simulink model "NarmaMotorNoDisrtub"  (R2019b)
settings: Solver=FixedStepAuto  StartTime=0.0  StopTime=30  FixedStep=0.001  RelTol=1e-3
libraries: neural x1, simulink x1
settings Model: Creator=Emanuel  LastModifiedBy=Emanuel

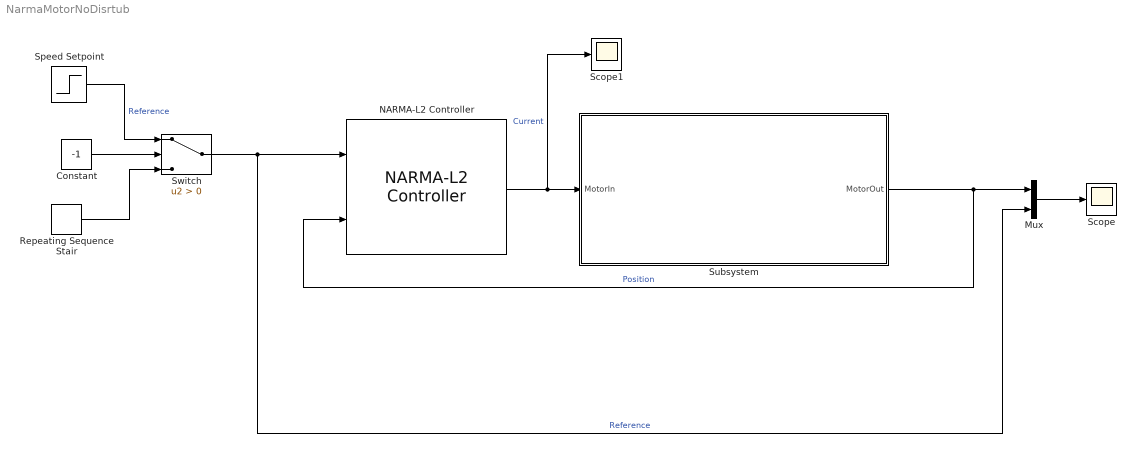
== system NarmaMotorNoDisrtub ==
  Constant : Constant  Value=-1
  Mux : Mux  Inputs=2
  NARMA-L2 Controller : neural/Control Systems/NARMA-L2 Controller  Normalize=0  IW1_1=[0.54422453296791495347 -8.2210065618848435776 -3.7830333244861606978 11.387541350251288108 3.5099764902727077498 -6.615636378792588701 10.270646774195714812 5.4834128974806324308 1.5686929425342031053 1.9741305625561031967 25.064932481428758848;10.05503986873957345 19.028606883106693459 11.182343981242496511 -2.8405339741589590297 -10.464572477682430929 -12.058389281694809725 -2.7714826032906860753 3.7461611803089196471 1.6204644865874766602 0.42415313297564860573 6.4827964395313486534;-335.44078668579430769 286.573015971562711 -187.68734927917793698 319.26608410688868389 221.01642027287860515 -305.40111344708714114 14.276828358611235004 9.9727003878624458366 6.7628793436236751546 9.1349517204525394476 14.179101495100859154;-1.7066174237370790312 -2.2638558722067476658 -2.7406505835762486889 -3.5321189662734870929 -6.5949213353093112389 -14.197286237901327155 2.2799959818071116047 4.0911747950291443843 2.9687832632498922791 3.416878733775998267 5.154880925569540473;-1.6730363884494878768 -5.4151164756102057041 -4.3929057393414607802 -8.1743670020292746869 2.9188688371473987537 18.969447318711061712 -8.529293132078448636 -14.164467720173188781 -10.587852748498855604 -13.551691179760860351 -17.974918470746633403;-3.2591311314982274183 12.337883279114715052 3.2937395594010450139 -30.11284141382879298 32.397534092837638298 -14.32400266854321913 -130.88652771808443731 140.69912550368584903 374.98954455414616405 -459.99858877533671375 -38.476614441129676436]  IW3_2=[-2.7577965784019937701 1.2752231451468867274 1.3996074068349657615 1.2105704890023423204 0.45470321325507695454 -1.2832715227445807837 -0.56158279430395419141 0.37486869307057324452 0.21875572119050948339 0.26450832397968576659 0.77097807764282566545;48.743457576208506055 -5.1531631914190034749 87.065999962059905215 -130.80082279171415394 -103.01087375687944814 97.749403698778010607 71.782150931217856282 55.062621026612909247 42.342961685691626883 43.689160160536054889 47.863257581946839991;5.4573369611260131862 0.22021020308996286374 -24.481423723828033445 -19.157095519588718702 14.135516604963051179 22.874994686256922449 -12.957341738873221715 -3.2165777199510738882 -4.3445828325806790104 -4.4947755060824272633 -3.6135327556077121436;488.07923945828918022 39.889515032705716635 -417.61236881668963861 -624.00642188413860367 371.51404644190978388 122.86999927681219447 -172.9512281008499599 322.0262465292354932 -249.15696488802083763 -274.34942750037879478 -268.53930455658172605;10.614257373293852993 -12.928226038048435953 1.8007341854585847685 0.47590664481989075618 1.3382033156911337102 11.791127023375008065 -1.4570318424168127169 6.6858980619533374679 0.99572516274640121559 3.596724941205785786 5.2562534427693412553;39.573323685332226773 -89.563598565790471184 68.345044595284250022 29.624767071379650929 -64.693171197386988069 16.751714047732363611 9.8626289348993783079 17.769837346136569067 -36.363423331338900368 -48.550247810202122878 -46.730060307809090148]  IW5_3=2.3941954495172454997  LW2_1=[-23.095405534712167395 -2.6857105544596406865 -21.818814964827854652 59.319651534505496215 -14.990739595435632836 11.470481340866285791]  LW4_3=[16.985094766801438482 -4.5039267178616082532 11.682340792277063457 -12.70858501600824475 29.633912642875980481 -6.7500019987399628718]  LW5_4=24.134279084852479969  LW6_5=0.037657415187600851159  LW6_2=-24.147602895572209292  B1=[-4.713627645162457469;-3.0956134780243815818;-958.89880089222197057;0.66118087049018392509;2.3947070143521007601;-54.856652664170525213]  B2=-90.876737356172270665  B3=[1.8381314321633948072;-17.367269795865190929;-1.6971158466136648801;23.48024490677872933;0.91873759677855559858;7.5471221598972650924]  B4=25.815736611914807952  Limit_output=0  min_output=-Inf  max_output=Inf  Use_Previous_Weights=1  Ts=0.05  S1=6  Ni=6  Nj=6  sim_file=SoleModelNoDistrubance  trainfun=trainlm  Use_validation=1  Use_Testing=1  max_i=40  min_i=1  max_i_int=4  min_i_int=2  sam_training=10000  epochs=500  minp=1.2838861864609374397  maxp=39.753006491435613157  mint=2000.3866487334141766  maxt=39.753006491435613157
      settings: SourceProductName=Deep Learning Toolbox  SourceProductBaseCode=NN
  Repeating Sequence Stair : simulink/Sources/Repeating Sequence Stair  OutValues=[1000 2000 3000 4000 5000].'  tsamp=4  OutMin=[]  OutMax=[]  OutDataTypeStr=double  OutputDataTypeScalingMode=double  OutDataType=fixdt(0,8)  ConRadixGroup=Best Precision: Vector-wise  OutScaling=2^-12
  Scope : Scope
  Scope1 : Scope
  Speed Setpoint : Step  Time=5  Before=2000  After=3000  SampleTime=0
  Subsystem : Subsystem
  Switch : Switch  Criteria=u2 > Threshold
  wires:
  NARMA-L2 Controller/1 -> Scope1/1, Subsystem/1(MotorIn)  "Current"
  Subsystem/1("MotorOut ") -> NARMA-L2 Controller/2, Mux/1  "Position"
  Mux/1 -> Scope/1
  Switch/1 -> Mux/2, NARMA-L2 Controller/1  "Reference"
  Repeating Sequence Stair/1 -> Switch/3
  Speed Setpoint/1 -> Switch/1  "Reference"
  Constant/1 -> Switch/2

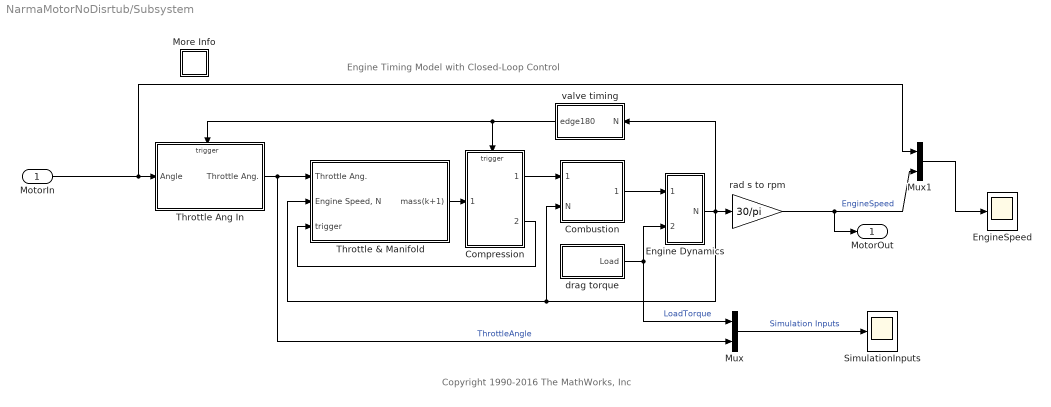
== system NarmaMotorNoDisrtub/Subsystem ==
  note: Copyright 1990-2016 The MathWorks, Inc
  note: Engine Timing Model with Closed-Loop Control
  MotorIn : Inport
  Combustion : Subsystem
  Compression : Subsystem  TreatAsAtomicUnit=on
  Engine Dynamics : Subsystem
  EngineSpeed : Scope
  More Info : Subsystem
      settings: OpenFcn=showdemo(bdroot(gcb))
      mask Display: disp('?')
  Mux : Mux  Inputs=2
  Mux1 : Mux  Inputs=2
  SimulationInputs : Scope
  Throttle & Manifold : Subsystem
  Throttle Ang In : Subsystem  TreatAsAtomicUnit=on
  drag torque : Subsystem
  rad s to rpm : Gain  Gain=30/pi  SaturateOnIntegerOverflow=on  OutDataTypeStr=Inherit: Same as input  ParamDataTypeStr=Inherit: Same as input
  valve timing : Subsystem
  "MotorOut " : Outport
  wires:
  Combustion/1(Torque) -> Engine Dynamics/1(Teng)
  Throttle Ang In/1(Throttle Ang.) -> Mux/2, Throttle & Manifold/1(Throttle Ang.)  "ThrottleAngle"
  drag torque/1(Load) -> Mux/1, Engine Dynamics/2(Tload)  "LoadTorque"
  MotorIn/1 -> Mux1/1, Throttle Ang In/1(Angle)
  Throttle & Manifold/1(mass(k+1)) -> Compression/1(mass(k+1))
  Compression/2(trigger) -> Throttle & Manifold/3(trigger)
  Mux/1 -> SimulationInputs/1  "Simulation Inputs"
  rad s to rpm/1 -> "MotorOut "/1, Mux1/2  "EngineSpeed"
  Compression/1(mass(k)) -> Combustion/1(Air Charge)
  Mux1/1 -> EngineSpeed/1
  valve timing/1(edge180) -> Throttle Ang In/Trigger, Compression/Trigger
  Engine Dynamics/1(N) -> rad s to rpm/1, valve timing/1(N), Throttle & Manifold/2("Engine Speed, N"), Combustion/2(N)

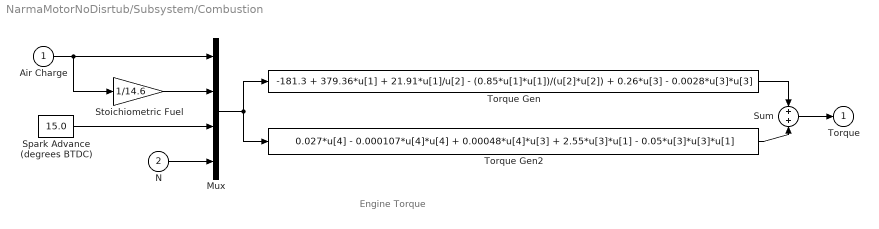
== system NarmaMotorNoDisrtub/Subsystem/Combustion ==
  note: Engine Torque
  Air Charge : Inport
  N : Inport  Port=2
  Mux : Mux
  Spark Advance (degrees BTDC) : Constant  Value=15.0
  Stoichiometric Fuel : Gain  Gain=1/14.6  SaturateOnIntegerOverflow=on  OutDataTypeStr=Inherit: Same as input  ParamDataTypeStr=Inherit: Same as input
  Sum : Sum  SaturateOnIntegerOverflow=on  InputSameDT=on  OutDataTypeStr=Inherit: Same as first input
  Torque Gen : Fcn  Expr=-181.3 + 379.36*u[1] + 21.91*u[1]/u[2] - (0.85*u[1]*u[1])/(u[2]*u[2]) + 0.26*u[3] - 0.0028*u[3]*u[3]
  Torque Gen2 : Fcn  Expr=0.027*u[4] - 0.000107*u[4]*u[4] + 0.00048*u[4]*u[3] + 2.55*u[3]*u[1] - 0.05*u[3]*u[3]*u[1]
  Torque : Outport  InitialOutput=0
  wires:
  Stoichiometric Fuel/1 -> Mux/2
  Spark Advance (degrees BTDC)/1 -> Mux/3
  N/1 -> Mux/4
  Air Charge/1 -> Stoichiometric Fuel/1, Mux/1
  Mux/1 -> Torque Gen/1, Torque Gen2/1
  Torque Gen2/1 -> Sum/2
  Torque Gen/1 -> Sum/1
  Sum/1 -> Torque/1

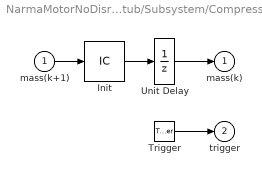
== system NarmaMotorNoDisrtub/Subsystem/Compression ==
  mass(k+1) : Inport
  Trigger : TriggerPort  TriggerType=either  VariantControl=Variant  ShowOutputPort=on
  Init : InitialCondition  Value=0.152
  Unit Delay : UnitDelay  InitialCondition=0.152  SampleTime=-1  HasFrameUpgradeWarning=on
  mass(k) : Outport  InitialOutput=0.152
  trigger : Outport  Port=2  InitialOutput=-1
  wires:
  Init/1 -> Unit Delay/1
  mass(k+1)/1 -> Init/1
  Unit Delay/1 -> mass(k)/1
  Trigger/1 -> trigger/1

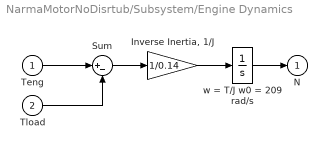
== system NarmaMotorNoDisrtub/Subsystem/Engine Dynamics ==
  Teng : Inport
  Tload : Inport  Port=2
  "Inverse Inertia, 1/J" : Gain  Gain=1/0.14  SaturateOnIntegerOverflow=on  OutDataTypeStr=Inherit: Same as input  ParamDataTypeStr=Inherit: Same as input
  Sum : Sum  Inputs=|+-  SaturateOnIntegerOverflow=on  InputSameDT=on  OutDataTypeStr=Inherit: Same as first input
  w = T/J w0 = 209 rad/s : Integrator  InitialCondition=209.48
  N : Outport  InitialOutput=0
  wires:
  "Inverse Inertia, 1/J"/1 -> w = T/J w0 = 209 rad/s/1
  w = T/J w0 = 209 rad/s/1 -> N/1
  Sum/1 -> "Inverse Inertia, 1/J"/1
  Teng/1 -> Sum/1
  Tload/1 -> Sum/2

== system NarmaMotorNoDisrtub/Subsystem/More Info ==

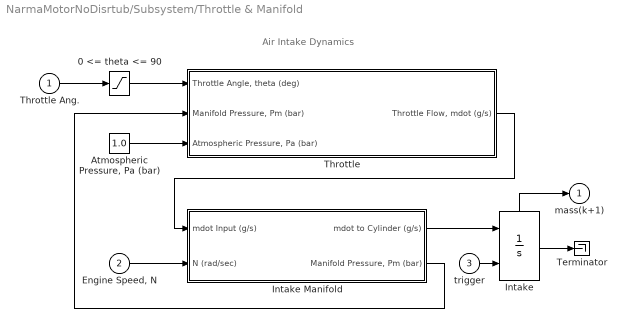
== system NarmaMotorNoDisrtub/Subsystem/Throttle & Manifold ==
  note: Air Intake Dynamics
  Throttle Ang. : Inport
  "Engine Speed, N" : Inport  Port=2
  trigger : Inport  Port=3
  0 <= theta <= 90 : Saturate  UpperLimit=90  LowerLimit=0
  "Atmospheric Pressure, Pa (bar)" : Constant  Value=1.0
  Intake : Integrator  ExternalReset=either  ShowStatePort=on
  Intake Manifold : Subsystem
  Terminator : Terminator
  Throttle : Subsystem
  mass(k+1) : Outport  InitialOutput=0
  wires:
  0 <= theta <= 90/1 -> Throttle/1("Throttle Angle, theta (deg)")
  Throttle Ang./1 -> 0 <= theta <= 90/1
  Throttle/1("Throttle Flow, mdot (g/s)") -> Intake Manifold/1(mdot Input (g/s))
  "Engine Speed, N"/1 -> Intake Manifold/2(N (rad/sec))
  Intake Manifold/2("Manifold Pressure, Pm (bar)") -> Throttle/2("Manifold Pressure, Pm (bar)")
  Intake Manifold/1(mdot to Cylinder (g/s)) -> Intake/1
  "Atmospheric Pressure, Pa (bar)"/1 -> Throttle/3("Atmospheric Pressure, Pa (bar) ")
  Intake/State -> mass(k+1)/1
  trigger/1 -> Intake/2
  Intake/1 -> Terminator/1

== system NarmaMotorNoDisrtub/Subsystem/Throttle Ang In ==
  note: Controller Subsystem
  Angle : Inport
  Trigger : TriggerPort  TriggerType=either  VariantControl=Variant
  Throttle Ang. : Outport  InitialOutput=8.973
  wires:
  Angle/1 -> Throttle Ang./1

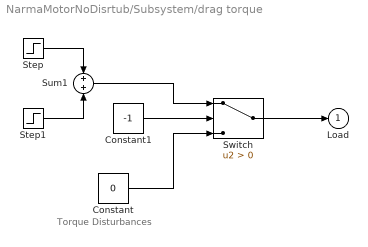
== system NarmaMotorNoDisrtub/Subsystem/drag torque ==
  note: Torque Disturbances
  Constant : Constant  Value=0
  Constant1 : Constant  Value=-1
  Step : Step  Time=2  Before=25  After=20  SampleTime=0
  Step1 : Step  Time=8  After=5  SampleTime=0
  Sum1 : Sum  SaturateOnIntegerOverflow=on  InputSameDT=on  OutDataTypeStr=Inherit: Same as first input
  Switch : Switch  Criteria=u2 > Threshold
  Load : Outport  InitialOutput=0
  wires:
  Sum1/1 -> Switch/1
  Step/1 -> Sum1/1
  Step1/1 -> Sum1/2
  Switch/1 -> Load/1
  Constant/1 -> Switch/3
  Constant1/1 -> Switch/2

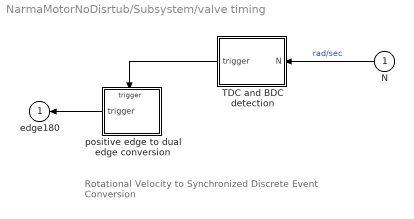
== system NarmaMotorNoDisrtub/Subsystem/valve timing ==
  note: Rotational Velocity to Synchronized
      | Discrete Event Conversion
  N : Inport
  TDC and BDC detection : Subsystem
  positive edge to dual edge conversion : Subsystem  TreatAsAtomicUnit=on
  edge180 : Outport  InitialOutput=-1
  wires:
  TDC and BDC detection/1(trigger) -> positive edge to dual edge conversion/Trigger
  positive edge to dual edge conversion/1(trigger) -> edge180/1
  N/1 -> TDC and BDC detection/1(N)  "rad/sec"

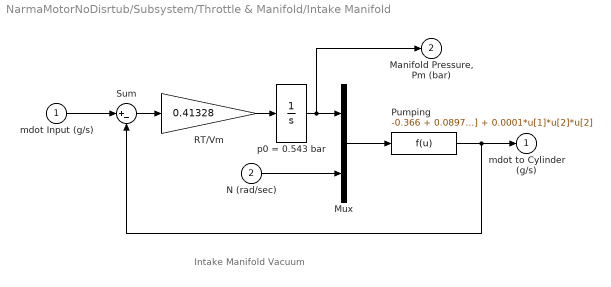
== system NarmaMotorNoDisrtub/Subsystem/Throttle & Manifold/Intake Manifold ==
  note: Intake Manifold Vacuum
  mdot Input (g/s) : Inport
  N (rad/sec) : Inport  Port=2
  Mux : Mux  Inputs=2
  Pumping : Fcn  Expr=-0.366 + 0.08979*u[1]*u[2] - 0.0337*u[2]*u[1]*u[1] + 0.0001*u[1]*u[2]*u[2]
  RT/Vm : Gain  Gain=0.41328  SaturateOnIntegerOverflow=on  OutDataTypeStr=Inherit: Same as input  ParamDataTypeStr=Inherit: Same as input
  Sum : Sum  Inputs=|+-  SaturateOnIntegerOverflow=on  InputSameDT=on  OutDataTypeStr=Inherit: Same as first input
  p0 = 0.543 bar : Integrator  InitialCondition=.543
  mdot to Cylinder (g/s) : Outport  InitialOutput=0
  "Manifold Pressure, Pm (bar)" : Outport  Port=2  InitialOutput=0
  wires:
  mdot Input (g/s)/1 -> Sum/1
  RT/Vm/1 -> p0 = 0.543 bar/1
  N (rad/sec)/1 -> Mux/2
  Mux/1 -> Pumping/1
  p0 = 0.543 bar/1 -> Mux/1, "Manifold Pressure, Pm (bar)"/1
  Sum/1 -> RT/Vm/1
  Pumping/1 -> Sum/2, mdot to Cylinder (g/s)/1

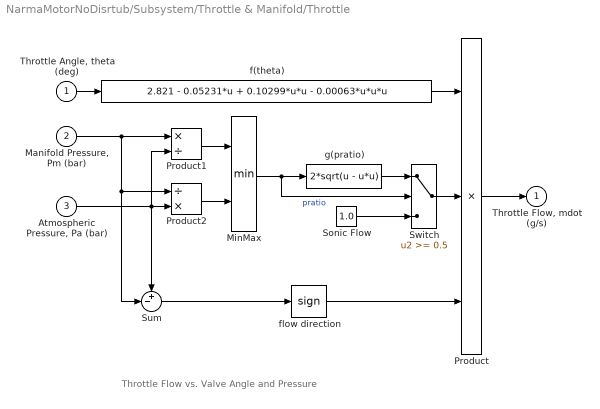
== system NarmaMotorNoDisrtub/Subsystem/Throttle & Manifold/Throttle ==
  note: Throttle Flow vs. Valve Angle and Pressure
  "Throttle Angle, theta (deg)" : Inport
  "Manifold Pressure, Pm (bar)" : Inport  Port=2
  "Atmospheric Pressure, Pa (bar) " : Inport  Port=3
  MinMax : MinMax  Inputs=2  SaturateOnIntegerOverflow=on  InputSameDT=on
  Product : Product  Inputs=3  SaturateOnIntegerOverflow=on  RndMeth=Zero  InputSameDT=on  OutDataTypeStr=Inherit: Same as first input
  Product1 : Product  Inputs=*/  SaturateOnIntegerOverflow=on  RndMeth=Zero  InputSameDT=on  OutDataTypeStr=Inherit: Same as first input
  Product2 : Product  Inputs=/*  SaturateOnIntegerOverflow=on  RndMeth=Zero  InputSameDT=on  OutDataTypeStr=Inherit: Same as first input
  "Sonic Flow " : Constant  Value=1.0
  Sum : Sum  Inputs=+-|  SaturateOnIntegerOverflow=on  InputSameDT=on  OutDataTypeStr=Inherit: Same as first input
  Switch : Switch  Threshold=0.5  SaturateOnIntegerOverflow=on  InputSameDT=on
  f(theta) : Fcn  Expr=2.821 - 0.05231*u + 0.10299*u*u - 0.00063*u*u*u
  flow direction : Signum
  g(pratio) : Fcn  Expr=2*sqrt(u - u*u)
  "Throttle Flow, mdot (g/s)" : Outport  InitialOutput=0
  wires:
  "Manifold Pressure, Pm (bar)"/1 -> Sum/2, Product2/1, Product1/1
  Product2/1 -> MinMax/2
  Product1/1 -> MinMax/1
  "Atmospheric Pressure, Pa (bar) "/1 -> Sum/1, Product2/2, Product1/2
  g(pratio)/1 -> Switch/1
  "Sonic Flow "/1 -> Switch/3
  Switch/1 -> Product/2
  flow direction/1 -> Product/3
  Sum/1 -> flow direction/1
  MinMax/1 -> Switch/2, g(pratio)/1  "pratio"
  "Throttle Angle, theta (deg)"/1 -> f(theta)/1
  Product/1 -> "Throttle Flow, mdot (g/s)"/1
  f(theta)/1 -> Product/1

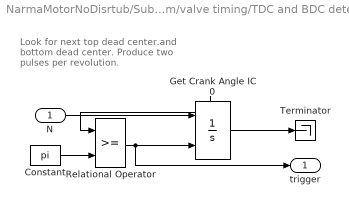
== system NarmaMotorNoDisrtub/Subsystem/valve timing/TDC and BDC detection ==
  note: Look for next top dead center.and
      | bottom dead center.
      | Produce two pulses per revolution.
  N : Inport
  Constant : Constant  Value=pi
  Get Crank Angle IC 0 : Integrator  ExternalReset=rising  ShowStatePort=on
  Relational Operator : RelationalOperator  OutDataTypeStr=boolean  RndMeth=Nearest  InputSameDT=on
  Terminator : Terminator
  trigger : Outport  InitialOutput=0
  wires:
  N/1 -> Get Crank Angle IC 0/1
  Relational Operator/1 -> trigger/1, Get Crank Angle IC 0/2
  Constant/1 -> Relational Operator/2
  Get Crank Angle IC 0/State -> Relational Operator/1
  Get Crank Angle IC 0/1 -> Terminator/1

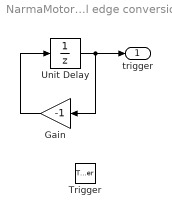
== system NarmaMotorNoDisrtub/Subsystem/valve timing/positive edge to dual edge conversion ==
  Trigger : TriggerPort  VariantControl=Variant
  Gain : Gain  Gain=-1  SaturateOnIntegerOverflow=on  OutDataTypeStr=Inherit: Same as input  ParamDataTypeStr=Inherit: Same as input
  Unit Delay : UnitDelay  InitialCondition=1  SampleTime=-1  HasFrameUpgradeWarning=on
  trigger : Outport  InitialOutput=-1
  wires:
  Gain/1 -> Unit Delay/1
  Unit Delay/1 -> trigger/1, Gain/1
